simulink model "xmenora0nolubricado"  (R2022a)
settings: Solver=VariableStepAuto  StartTime=0.0  StopTime=10.0  RelTol=1e-3
settings Model: Creator=melaaa  LastModifiedBy=melaaa

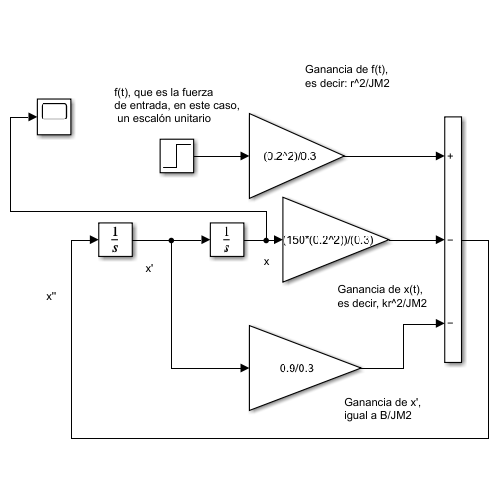
[thumbnail: Simulink's stored preview of the top-level diagram]
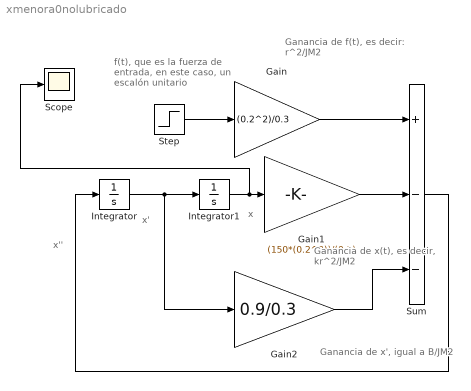
== system xmenora0nolubricado ==
  note: x
  note: x'
  note: x''
  note: Ganancia de x',
      | igual a B/JM2
  note: Ganancia de x(t),
      | es decir, kr^2/JM2
  note: Ganancia de f(t),
      | es decir: r^2/JM2
  note: f(t), que es la fuerza
      | de entrada, en este caso,
      |  un escalón unitario
  Gain : Gain  Gain=(0.2^2)/0.3
  Gain1 : Gain  Gain=(150*(0.2^2))/(0.3)
  Gain2 : Gain  Gain=0.9/0.3
  Integrator : Integrator
  Integrator1 : Integrator
  Scope : Scope
  Step : Step  Time=0  SampleTime=0
  Sum : Sum  Inputs=+--
  wires:
  Integrator/1 -> Gain2/1, Integrator1/1
  Step/1 -> Gain/1
  Gain/1 -> Sum/1
  Gain1/1 -> Sum/2
  Gain2/1 -> Sum/3
  Sum/1 -> Integrator/1
  Integrator1/1 -> Scope/1, Gain1/1
